simulink model "sourceLocalization"  (R2020a)
settings: Solver=VariableStepAuto  StartTime=0.0  StopTime=inf  RelTol=1e-3
model workspace (MAT data in the model file):
  VADThreshold = 0.85
  frameLength = 10000
  fs = 44100
undefined symbols (not defined in the file or in its folder): phased
libraries: dspsnks4 x1, dspsrcs4 x1, dspvision x1, phaseddoalib x1, dspnetwork x1, audiomeasurements x1
settings Model: OrderedModelArguments=off  Creator=GH  LastModifiedBy=GH

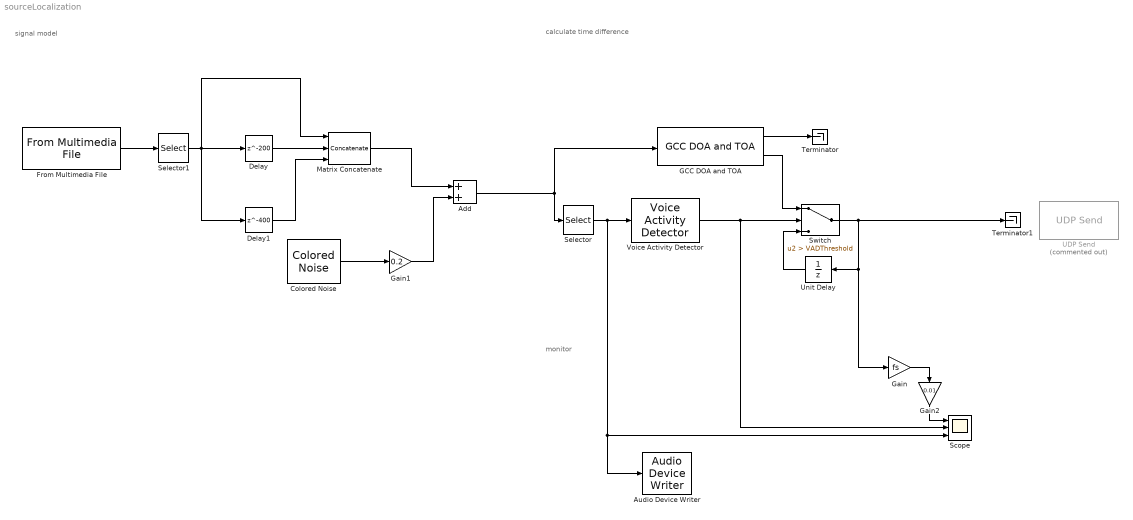
== system sourceLocalization ==
  note: monitor
  note: calculate time difference
  note: signal model
  Add : Sum
  Audio Device Writer : dspsnks4/Audio Device Writer  Driver=DirectSound  Device=Default  InheritSampleRate=on  SampleRate=44100  BitDepth=16-bit integer  BufferSize=4096  NumBuffers=10  DefaultOutputChannelMapping=on  OutputChannelMapping=1:2  OutputNumUnderrunSamples=off  DriverIdx=1  DeviceWarnFlag=''
  Colored Noise : dspsrcs4/Colored Noise  Color=pink  InverseFrequencyPower=1  BoundedOutput=on  NumChannels=3  OutputDataType=double  SamplesPerFrame=frameLength  SampleTime=1/fs  RandomStream=mt19937ar with seed  Seed=67  SimulateUsing=Interpreted execution
      settings: SourceProductBaseCode=DS
  Delay : Delay  DelayLength=200  InputProcessing=Columns as channels (frame based)  UseCircularBuffer=on
  Delay1 : Delay  DelayLength=400  InputProcessing=Columns as channels (frame based)  UseCircularBuffer=on
  From Multimedia File : dspvision/From Multimedia File  inputFilename=D:\Files\Research\1a 其他\测试用音频\美谈不美repair.wav  readRange=[1 Inf]  loop=on  numPlays=inf  outputStreams=Audio only  videoDataType=single  audioDataType=double  inheritSampleTime=on  userDefinedSampleTime=1/30  noAudioOutput=off  isIntensityVideo=off  fourcc=RGB  colorVideoFormat=Separate color signals  outputEOF=off  dataOrg=Column-major  audioFrameSize=frameLength  computeAudioFrameSize=off  outSamplingMode=Sample based
  GCC DOA and TOA : phaseddoalib/GCC DOA and TOA  PropagationSpeed=300  SampleRateFromInputCheckbox=on  SampleRate=1e6  SensorPairSource=Auto  SensorPair=[ 2; 1 ]  CorrelationOutputPort=off  DelayOutputPort=on  SimulateUsing=Interpreted execution  SensorArray=phased.ULA('NumElements',3,'Element',phased.OmnidirectionalMicrophoneElement(),'ElementSpacing',200/44100/sind(12)*300,'ArrayAxis','x')
      settings: SourceProductBaseCode=AR
  Gain : Gain  Gain=fs
  Gain1 : Gain  Gain=0.2
  Gain2 : Gain  Gain=0.01
  Matrix Concatenate : Concatenate  NumInputs=3  Mode=Multidimensional array  ConcatenateDimension=2
  Scope : Scope  NumInputPorts=3
  Selector : Selector  NumberOfDimensions=2  InputPortWidth=3  IndexOptions=Select all,Index vector (dialog)  Indices=[1 3],1  OutputSizes=1,1
  Selector1 : Selector  NumberOfDimensions=2  InputPortWidth=3  IndexOptions=Select all,Index vector (dialog)  Indices=[1 3],1  OutputSizes=1,1
  Switch : Switch  Criteria=u2 > Threshold  Threshold=VADThreshold
  Terminator : Terminator
  Terminator1 : Terminator
  UDP Send : dspnetwork/UDP Send  Commented=on  remoteURL='127.0.0.1'  remotePort=25000  localURL='0.0.0.0'  localPortSource=Automatically determine  localPort=-1  sendBufferSize=8192  sampletime=-1  blockPlatform=[]  separateLengthPort=0
  Unit Delay : UnitDelay  InputProcessing=Columns as channels (frame based)  SampleTime=-1  HasFrameUpgradeWarning=on
  Voice Activity Detector : audiomeasurements/Voice Activity Detector  InputDomain=Time  Window=Hann  SidelobeAttenuation=60  InheritFFTLength=on  FFTLength=1024  SilenceToSpeechProbabilityPort=off  SilenceToSpeechProbability=0.2  SpeechToSilenceProbabilityPort=off  SpeechToSilenceProbability=0.1  OutputNoiseVariance=off  SimulateUsing=Code generation
      settings: SourceProductBaseCode=AU
  wires:
  From Multimedia File/1 -> Selector1/1
  Delay/1 -> Matrix Concatenate/2
  Delay1/1 -> Matrix Concatenate/3
  GCC DOA and TOA/1 -> Terminator/1
  Add/1 -> GCC DOA and TOA/1, Selector/1
  Voice Activity Detector/1 -> Scope/2, Switch/2
  GCC DOA and TOA/2 -> Switch/1
  Switch/1 -> Terminator1/1, Unit Delay/1, Gain/1
  Gain/1 -> Gain2/1
  Unit Delay/1 -> Switch/3
  Selector1/1 -> Matrix Concatenate/1, Delay1/1, Delay/1
  Colored Noise/1 -> Gain1/1
  Matrix Concatenate/1 -> Add/1
  Gain1/1 -> Add/2
  Gain2/1 -> Scope/1
  Selector/1 -> Audio Device Writer/1, Scope/3, Voice Activity Detector/1
